simulink model "EV_tracking"  (R2015a)
settings: Solver=ode3  StartTime=0.0  StopTime=10  FixedStep=1e-4  RelTol=1e-3
values from neighbouring files (symbols this model uses):
  B = 11.43    [Kanon_data.m]
  bf = b*f    (= 260)    [main.m]
  C = 1.314    [Kanon_data.m]
  car1 = 10    [main.m]
  car2 = 0    [main.m]
  Dref = 5    [main.m]
  J = 1.24    [Kanon_data.m]
  m = 800    [Kanon_data.m]
  N = m*g    (= 7840)    [Kanon_data.m]
  r = 0.32    [Kanon_data.m]
  tau = 0.2    [main.m]
undefined symbols (not defined in the file or in its folder): Kb, Ki, Kp, Tmax, Tmin
libraries: simulink x1
settings Model: Creator=yoshi  LastModifiedBy=yoshi

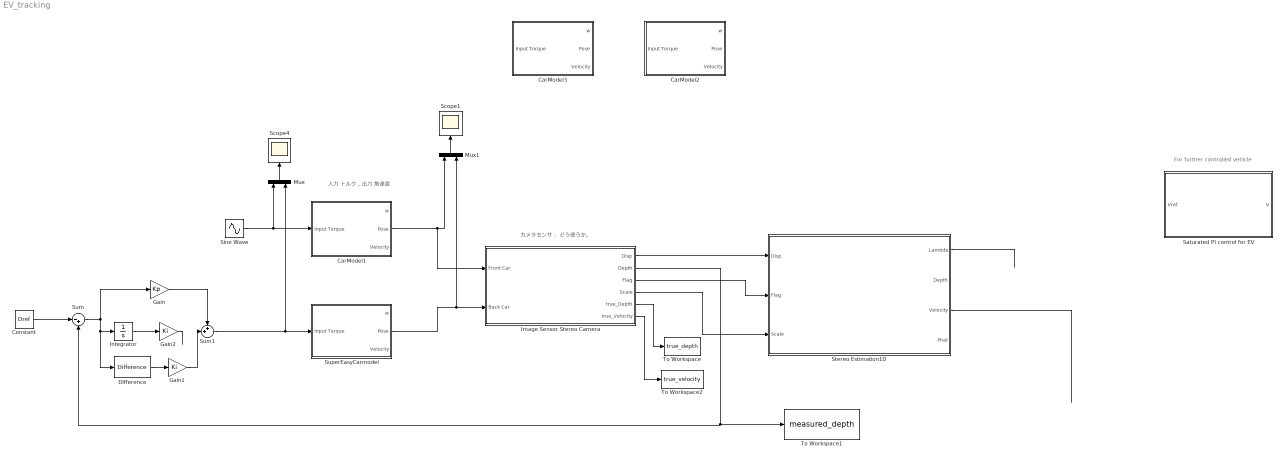
== system EV_tracking ==
  note: For further controlled vehicle
  note: 入力 トルク，出力 角速度
  note: カメラセンサ： どう使うか。
  CarModel1 : Subsystem
  CarModel2 : Subsystem
  CarModel3 : Subsystem
  Constant : Constant  Value=Dref
  Difference : simulink/Discrete/Difference  ICPrevInput=0.0  InputProcessing=Inherited  OutMin=[]  OutMax=[]  OutDataType=fixdt(1, 16)  OutScaling=2^-10  DoSatur=off
  Gain : Gain  Gain=Kp
  Gain1 : Gain  Gain=Ki
  Gain2 : Gain  Gain=Ki
  Image Sensor Stereo Camera : Subsystem
  Integrator : Integrator
  Mux : Mux  Inputs=2
  Mux1 : Mux  Inputs=2
  Saturated PI control for EV : Subsystem
  Scope1 : Scope
      settings: YMin=18  YMax=30  Decimation=10
  Scope4 : Scope
      settings: YMin=-12500  YMax=30000  SaveName=ScopeData5  Decimation=10
  Sine Wave : Sin  Amplitude=50  Bias=100  Frequency=0.2  SampleTime=0
  Stereo Estimation1D : MATLAB Function  TreatAsAtomicUnit=on
  Sum : Sum  Inputs=|-+
  Sum1 : Sum  Inputs=++|
  SuperEasyCarmodel : Subsystem
  To Workspace : ToWorkspace  VariableName=true_depth  SaveFormat=Timeseries  SampleTime=-1
  To Workspace1 : ToWorkspace  VariableName=measured_depth  SaveFormat=Timeseries  SampleTime=-1
  To Workspace2 : ToWorkspace  VariableName=true_velocity  SaveFormat=Timeseries  SampleTime=-1
  wires:
  Image Sensor Stereo Camera/1(Disp) -> Stereo Estimation1D/1(Disp)
  Image Sensor Stereo Camera/4(Scale) -> Stereo Estimation1D/3(Scale)
  Image Sensor Stereo Camera/3(Flag) -> Stereo Estimation1D/2(Flag)
  Stereo Estimation1D/1(Lambda) -> ?
  Stereo Estimation1D/3(Velocity) -> ?
  Sine Wave/1 -> CarModel1/1(Input Torque), Mux/1
  Integrator/1 -> Gain2/1
  Sum/1 -> Difference/1, Integrator/1, Gain/1
  Constant/1 -> Sum/1
  Gain2/1 -> ?
  Gain/1 -> Sum1/1
  Sum1/1 -> SuperEasyCarmodel/1(Input Torque), Mux/2
  Image Sensor Stereo Camera/5(true_Depth) -> To Workspace/1
  Image Sensor Stereo Camera/2(Depth) -> To Workspace1/1, Sum/2
  Mux/1 -> Scope4/1
  CarModel1/2(Pose) -> Mux1/1, Image Sensor Stereo Camera/1(Front Car)
  SuperEasyCarmodel/2(Pose) -> Mux1/2, Image Sensor Stereo Camera/2(Back Car)
  Mux1/1 -> Scope1/1
  Difference/1 -> Gain1/1
  Gain1/1 -> Sum1/2
  Image Sensor Stereo Camera/6(true_Velocity) -> To Workspace2/1

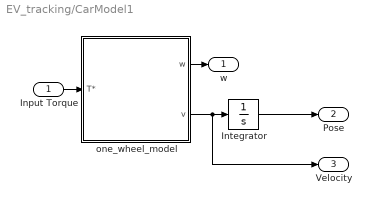
== system EV_tracking/CarModel1 ==
  Input Torque : Inport
  Integrator : Integrator  InitialCondition=car1
  one_wheel_model : Subsystem
  w : Outport
  Pose : Outport  Port=2
  Velocity : Outport  Port=3
  wires:
  Integrator/1 -> Pose/1
  one_wheel_model/1(w) -> w/1
  Input Torque/1 -> one_wheel_model/1(T*)
  one_wheel_model/2(v) -> Velocity/1, Integrator/1

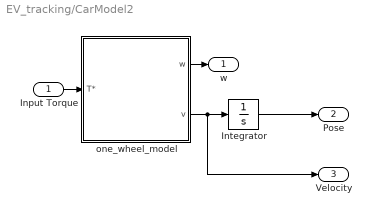
== system EV_tracking/CarModel2 ==
  Input Torque : Inport
  Integrator : Integrator  InitialCondition=car2
  one_wheel_model : Subsystem
  w : Outport
  Pose : Outport  Port=2
  Velocity : Outport  Port=3
  wires:
  one_wheel_model/2(v) -> Velocity/1, Integrator/1
  Input Torque/1 -> one_wheel_model/1(T*)
  one_wheel_model/1(w) -> w/1
  Integrator/1 -> Pose/1

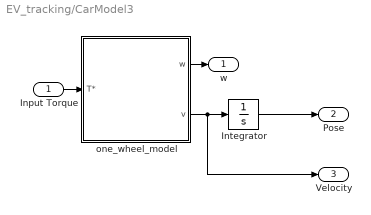
== system EV_tracking/CarModel3 ==
  Input Torque : Inport
  Integrator : Integrator  InitialCondition=car2
  one_wheel_model : Subsystem
  w : Outport
  Pose : Outport  Port=2
  Velocity : Outport  Port=3
  wires:
  one_wheel_model/2(v) -> Velocity/1, Integrator/1
  Input Torque/1 -> one_wheel_model/1(T*)
  one_wheel_model/1(w) -> w/1
  Integrator/1 -> Pose/1

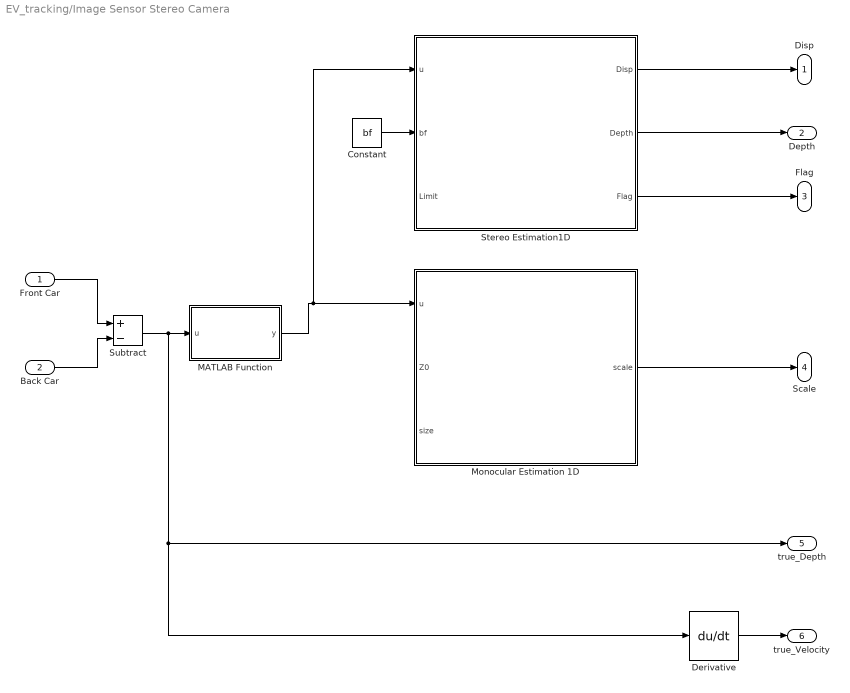
== system EV_tracking/Image Sensor Stereo Camera ==
  Front Car : Inport
  Back Car : Inport  Port=2
  Constant : Constant  Value=bf
  Derivative : Derivative
  MATLAB Function : MATLAB Function  TreatAsAtomicUnit=on
  Monocular Estimation 1D : MATLAB Function  TreatAsAtomicUnit=on
  Stereo Estimation1D : MATLAB Function  TreatAsAtomicUnit=on
  Subtract : Sum  Inputs=+-
  Disp : Outport
  Depth : Outport  Port=2
  Flag : Outport  Port=3
  Scale : Outport  Port=4
  true_Depth : Outport  Port=5
  true_Velocity : Outport  Port=6
  wires:
  MATLAB Function/1(y) -> Stereo Estimation1D/1(u), Monocular Estimation 1D/1(u)
  Stereo Estimation1D/1(Disp) -> Disp/1
  Stereo Estimation1D/3(Flag) -> Flag/1
  Stereo Estimation1D/2(Depth) -> Depth/1
  Constant/1 -> Stereo Estimation1D/2(bf)
  Monocular Estimation 1D/1(scale) -> Scale/1
  Back Car/1 -> Subtract/2
  Front Car/1 -> Subtract/1
  Subtract/1 -> Derivative/1, true_Depth/1, MATLAB Function/1(u)
  Derivative/1 -> true_Velocity/1

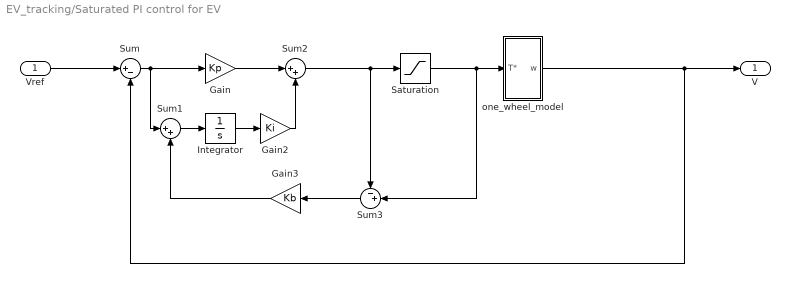
== system EV_tracking/Saturated PI control for EV ==
  Vref : Inport
  Gain : Gain  Gain=Kp
  Gain2 : Gain  Gain=Ki
  Gain3 : Gain  Gain=Kb
  Integrator : Integrator
  Saturation : Saturate  UpperLimit=Tmax  LowerLimit=Tmin
  Sum : Sum  Inputs=|+-
  Sum1 : Sum  Inputs=|++
  Sum2 : Sum  Inputs=|++
  Sum3 : Sum  Inputs=-+|
  one_wheel_model : Subsystem
  "V " : Outport
  wires:
  Sum/1 -> Sum1/1, Gain/1
  Gain3/1 -> Sum1/2
  Sum3/1 -> Gain3/1
  Sum1/1 -> Integrator/1
  Saturation/1 -> one_wheel_model/1(T*), Sum3/2
  Gain/1 -> Sum2/1
  Sum2/1 -> Saturation/1, Sum3/1
  Vref/1 -> Sum/1
  Gain2/1 -> Sum2/2
  one_wheel_model/1(w) -> "V "/1, Sum/2
  Integrator/1 -> Gain2/1

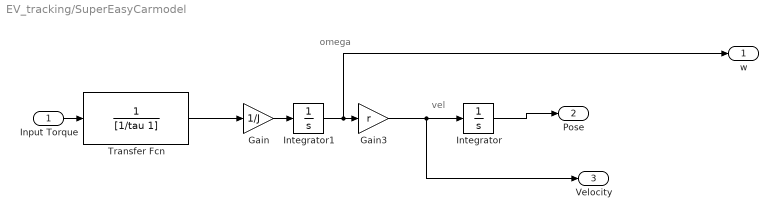
== system EV_tracking/SuperEasyCarmodel ==
  note: vel
  note: omega
  Input Torque : Inport
  Gain : Gain  Gain=1/J
  Gain3 : Gain  Gain=r
  Integrator : Integrator  InitialCondition=car2
  Integrator1 : Integrator
  Transfer Fcn : TransferFcn  Denominator=[1/tau 1]
  w : Outport
  Pose : Outport  Port=2
  Velocity : Outport  Port=3
  wires:
  Gain3/1 -> Velocity/1, Integrator/1
  Transfer Fcn/1 -> Gain/1
  Integrator1/1 -> w/1, Gain3/1
  Integrator/1 -> Pose/1
  Gain/1 -> Integrator1/1
  Input Torque/1 -> Transfer Fcn/1

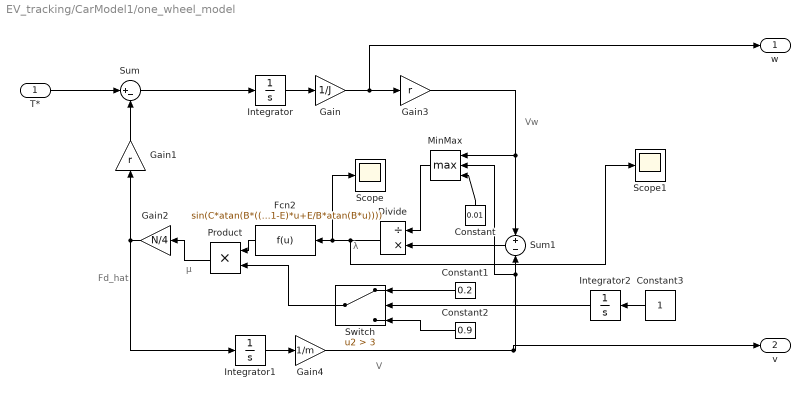
== system EV_tracking/CarModel1/one_wheel_model ==
  note: V
  note: Fd_hat
  note: Vw
  note: μ
  note: λ
  T* : Inport
  Constant : Constant  Value=0.01
  Constant1 : Constant  Value=0.2
  Constant2 : Constant  Value=0.9
  Constant3 : Constant
  Divide : Product  Inputs=/*
  Fcn2 : Fcn  Expr=sin(C*atan(B*((1-E)*u+E/B*atan(B*u))))
  Gain : Gain  Gain=1/J
  Gain1 : Gain  Gain=r
  Gain2 : Gain  Gain=N/4
  Gain3 : Gain  Gain=r
  Gain4 : Gain  Gain=1/m
  Integrator : Integrator
  Integrator1 : Integrator
  Integrator2 : Integrator
  MinMax : MinMax  Function=max  Inputs=3
  Product : Product
  Scope : Scope
  Scope1 : Scope
      settings: YMin=0.015  YMax=0.095  SaveName=ScopeData4
  Sum : Sum  Inputs=|+-
  Sum1 : Sum  Inputs=+|-
  Switch : Switch  Criteria=u2 > Threshold  Threshold=3
  w : Outport
  v : Outport  Port=2
  wires:
  Gain3/1 -> Sum1/1, MinMax/1
  Integrator2/1 -> Switch/2
  Constant3/1 -> Integrator2/1
  Constant2/1 -> Switch/3
  Switch/1 -> Product/2
  Product/1 -> Gain2/1
  Fcn2/1 -> Product/1
  Divide/1 -> Scope/1, Fcn2/1, Scope1/1
  MinMax/1 -> Divide/1
  Constant/1 -> MinMax/3
  Gain4/1 -> Sum1/2, MinMax/2, v/1
  Gain/1 -> Gain3/1, w/1
  Gain2/1 -> Integrator1/1, Gain1/1
  T*/1 -> Sum/1
  Constant1/1 -> Switch/1
  Gain1/1 -> Sum/2
  Sum1/1 -> Divide/2
  Integrator/1 -> Gain/1
  Integrator1/1 -> Gain4/1
  Sum/1 -> Integrator/1

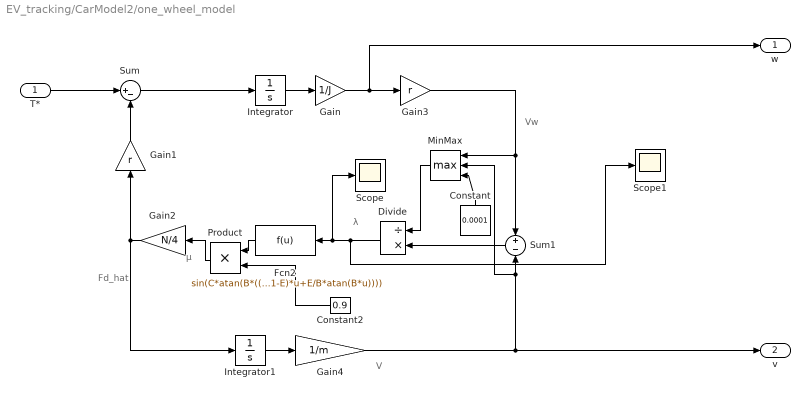
== system EV_tracking/CarModel2/one_wheel_model ==
  note: λ
  note: μ
  note: Vw
  note: Fd_hat
  note: V
  T* : Inport
  Constant : Constant  Value=0.0001
  Constant2 : Constant  Value=0.9
  Divide : Product  Inputs=/*
  Fcn2 : Fcn  Expr=sin(C*atan(B*((1-E)*u+E/B*atan(B*u))))
  Gain : Gain  Gain=1/J
  Gain1 : Gain  Gain=r
  Gain2 : Gain  Gain=N/4
  Gain3 : Gain  Gain=r
  Gain4 : Gain  Gain=1/m
  Integrator : Integrator
  Integrator1 : Integrator
  MinMax : MinMax  Function=max  Inputs=3
  Product : Product
  Scope : Scope
  Scope1 : Scope
      settings: YMin=0.015  YMax=0.095  SaveName=ScopeData4
  Sum : Sum  Inputs=|+-
  Sum1 : Sum  Inputs=+|-
  w : Outport
  v : Outport  Port=2
  wires:
  Sum/1 -> Integrator/1
  Integrator1/1 -> Gain4/1
  Integrator/1 -> Gain/1
  Sum1/1 -> Divide/2
  Gain1/1 -> Sum/2
  T*/1 -> Sum/1
  Gain2/1 -> Gain1/1, Integrator1/1
  Gain/1 -> w/1, Gain3/1
  Gain4/1 -> v/1, MinMax/2, Sum1/2
  Constant/1 -> MinMax/3
  MinMax/1 -> Divide/1
  Divide/1 -> Scope1/1, Fcn2/1, Scope/1
  Fcn2/1 -> Product/1
  Product/1 -> Gain2/1
  Gain3/1 -> MinMax/1, Sum1/1
  Constant2/1 -> Product/2

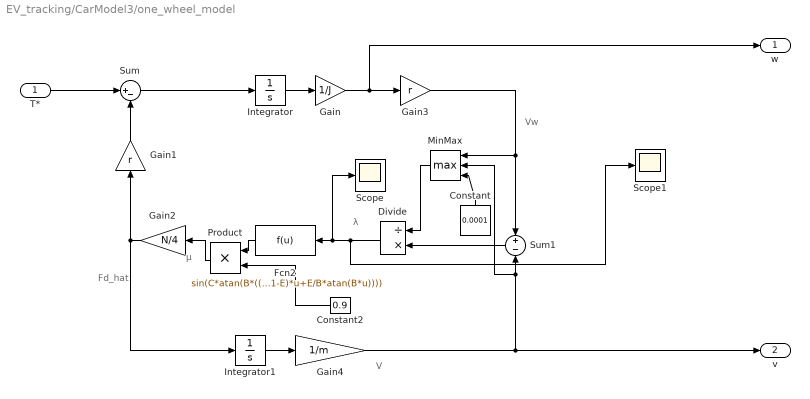
== system EV_tracking/CarModel3/one_wheel_model ==
  note: λ
  note: μ
  note: Vw
  note: Fd_hat
  note: V
  T* : Inport
  Constant : Constant  Value=0.0001
  Constant2 : Constant  Value=0.9
  Divide : Product  Inputs=/*
  Fcn2 : Fcn  Expr=sin(C*atan(B*((1-E)*u+E/B*atan(B*u))))
  Gain : Gain  Gain=1/J
  Gain1 : Gain  Gain=r
  Gain2 : Gain  Gain=N/4
  Gain3 : Gain  Gain=r
  Gain4 : Gain  Gain=1/m
  Integrator : Integrator
  Integrator1 : Integrator
  MinMax : MinMax  Function=max  Inputs=3
  Product : Product
  Scope : Scope
  Scope1 : Scope
      settings: YMin=0.015  YMax=0.095  SaveName=ScopeData4
  Sum : Sum  Inputs=|+-
  Sum1 : Sum  Inputs=+|-
  w : Outport
  v : Outport  Port=2
  wires:
  Sum/1 -> Integrator/1
  Integrator1/1 -> Gain4/1
  Integrator/1 -> Gain/1
  Sum1/1 -> Divide/2
  Gain1/1 -> Sum/2
  T*/1 -> Sum/1
  Gain2/1 -> Gain1/1, Integrator1/1
  Gain/1 -> w/1, Gain3/1
  Gain4/1 -> v/1, MinMax/2, Sum1/2
  Constant/1 -> MinMax/3
  MinMax/1 -> Divide/1
  Divide/1 -> Scope1/1, Fcn2/1, Scope/1
  Fcn2/1 -> Product/1
  Product/1 -> Gain2/1
  Gain3/1 -> MinMax/1, Sum1/1
  Constant2/1 -> Product/2

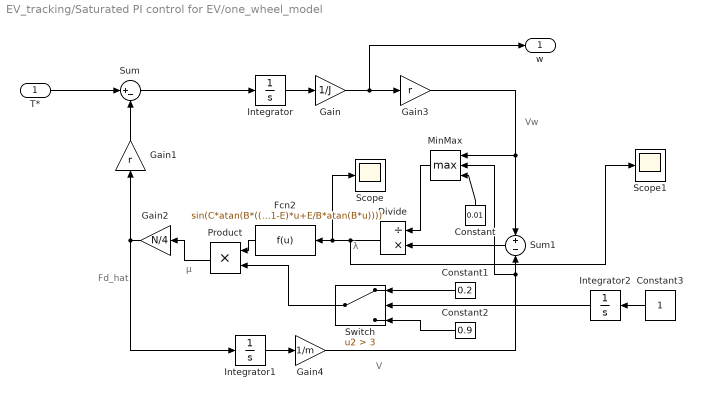
== system EV_tracking/Saturated PI control for EV/one_wheel_model ==
  note: λ
  note: μ
  note: Vw
  note: Fd_hat
  note: V
  T* : Inport
  Constant : Constant  Value=0.01
  Constant1 : Constant  Value=0.2
  Constant2 : Constant  Value=0.9
  Constant3 : Constant
  Divide : Product  Inputs=/*
  Fcn2 : Fcn  Expr=sin(C*atan(B*((1-E)*u+E/B*atan(B*u))))
  Gain : Gain  Gain=1/J
  Gain1 : Gain  Gain=r
  Gain2 : Gain  Gain=N/4
  Gain3 : Gain  Gain=r
  Gain4 : Gain  Gain=1/m
  Integrator : Integrator
  Integrator1 : Integrator
  Integrator2 : Integrator
  MinMax : MinMax  Function=max  Inputs=3
  Product : Product
  Scope : Scope
  Scope1 : Scope
      settings: YMin=0.015  YMax=0.095  SaveName=ScopeData4
  Sum : Sum  Inputs=|+-
  Sum1 : Sum  Inputs=+|-
  Switch : Switch  Criteria=u2 > Threshold  Threshold=3
  w : Outport
  wires:
  Sum/1 -> Integrator/1
  Integrator1/1 -> Gain4/1
  Integrator/1 -> Gain/1
  Sum1/1 -> Divide/2
  Gain1/1 -> Sum/2
  Constant1/1 -> Switch/1
  T*/1 -> Sum/1
  Gain2/1 -> Gain1/1, Integrator1/1
  Gain/1 -> w/1, Gain3/1
  Gain4/1 -> MinMax/2, Sum1/2
  Constant/1 -> MinMax/3
  MinMax/1 -> Divide/1
  Divide/1 -> Scope1/1, Fcn2/1, Scope/1
  Fcn2/1 -> Product/1
  Product/1 -> Gain2/1
  Switch/1 -> Product/2
  Constant2/1 -> Switch/3
  Constant3/1 -> Integrator2/1
  Integrator2/1 -> Switch/2
  Gain3/1 -> MinMax/1, Sum1/1

== matlab function EV_tracking/Image Sensor Stereo Camera/Monocular Estimation 1D ==
  data: u input; Z0 input; scale output; size input
function scale  = MonocularScale1D(u,Z0,size)
%#codegen

% Set 0.5m to be the reference depth
if nargin == 1
    Z0 = 0.5;
    size = 500;
end

scale = Z0/u;
Esize = size * scale + randn(1);
scale = Esize/size;
end

== matlab function EV_tracking/Image Sensor Stereo Camera/Stereo Estimation1D ==
  data: u input; bf input; Disp output; Limit input; Depth output; Flag output
function [Disp, Depth, Flag] = StereoCamera1D(u,bf,Limit)
%#codegen

% Set 0.5m to be the minimum depth
if nargin == 1
    Limit = 0.5;
    bf = 26; % 400*26  
else nargin == 2
    Limit = 0.5;
end

if u < Limit
    Flag = 0;
    Disp = 0;
    Depth = 0;
else 
    Disp = bf/u + randn(1); % add noise
    if Disp <= 0
        Disp = 0;
        Depth = 0;
        Flag = 0;
    else
        Depth = bf/Disp;
        Flag = 1;
    end
end

end

== matlab function EV_tracking/Image Sensor Stereo Camera/MATLAB Function ==
  data: u input; y output
function y = ColisionDetection(u)
%#codegen
if u < 0
  error('Collision Occured!!')
else
  y = u;
end

end

== matlab function EV_tracking/Stereo Estimation1D ==
  data: Disp input; Flag input; Lambda output; Scale input; Depth output; Velocity output; Phat output
function [Lambda, Depth, Velocity, Phat] = EKFfilter_ver1(Disp,Flag,Scale)
%#codegen

persistent X P start;
if isempty(X)
    X = [0 0 0]; 
    P =  diag([10000,10000,10000]);
    start = 0;
end

Lambda = X(1);
Depth = X(2);
Velocity = X(3);
Phat = P;
end
